simulink model "Closed_loop_Sim_2017a"  (R2017a)
settings: Solver=FixedStepAuto  StartTime=0.0  StopTime=400  FixedStep=tstep  RelTol=1e-3  EnableMultiTasking=on
InitFcn:
  | initSim;
values from neighbouring files (symbols this model uses):
  par = problem.data    [initSim.m]
undefined symbols (not defined in the file or in its folder): m, problem
settings Model: Creator=yn15  LastModifiedBy=Yuanb
settings OptimizationCC: LifeSpan=inf
settings DebuggingCC: SFUnexpectedBacktrackingDiag=warning  SFNoUnconditionalDefaultTransitionDiag=warning  SFExecutionAtInitializationDiag=none
settings GRTTargetCC: TargetLangStandard=C89/C90 (ANSI)
settings ConfigComp: CovMetricSettings=dw  CovHtmlReporting=on  CovSaveCumulativeToWorkspaceVar=on  CovSaveSingleToWorkspaceVar=on  CovExternalEMLEnable=off

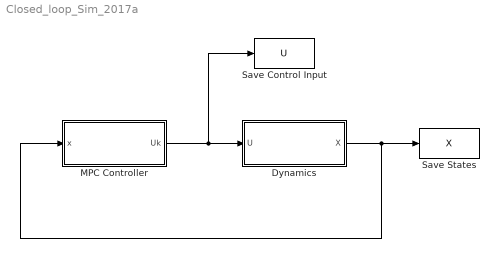
== system Closed_loop_Sim_2017a ==
  Dynamics : Subsystem
  "MPC Controller " : Subsystem
  Save Control Input : ToWorkspace  VariableName=U  SampleTime=-1
      settings: Save2DSignal=2-D array (concatenate along first dimension)
  Save States : ToWorkspace  VariableName=X  SampleTime=-1
  wires:
  "MPC Controller "/1(Uk) -> Dynamics/1(U), Save Control Input/1
  Dynamics/1(X) -> Save States/1, "MPC Controller "/1(x)

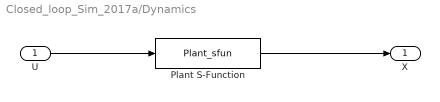
== system Closed_loop_Sim_2017a/Dynamics ==
  U : Inport
  Plant S-Function : S-Function  FunctionName=Plant_sfun  Parameters=par;problem.states.x0  SFunctionDeploymentMode=off  EnableBusSupport=off
  X : Outport
  wires:
  Plant S-Function/1 -> X/1
  U/1 -> Plant S-Function/1

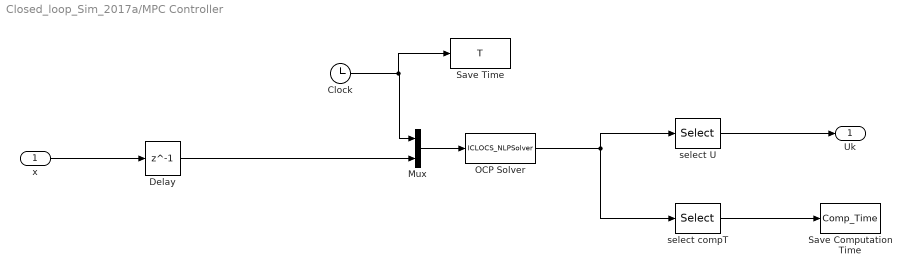
== system Closed_loop_Sim_2017a/MPC Controller  ==
  x : Inport
  Clock : Clock
  Delay : Delay  DelayLength=1  InitialCondition=[problem.states.x0]
  Mux : Mux  Inputs=2
  OCP Solver : MATLABFcn  MATLABFcn=ICLOCS_NLPSolver  OutputDimensions=m+2
  "Save Computation Time " : ToWorkspace  VariableName=Comp_Time  SampleTime=-1
      settings: Save2DSignal=2-D array (concatenate along first dimension)
  Save Time : ToWorkspace  VariableName=T  SampleTime=-1
      settings: Save2DSignal=2-D array (concatenate along first dimension)
  select U : Selector  IndexOptions=Index vector (dialog)  Indices=3:m+2  OutputSizes=1
  select compT : Selector  IndexOptions=Index vector (dialog)  Indices=2  OutputSizes=1
  Uk : Outport
  wires:
  select U/1 -> Uk/1
  x/1 -> Delay/1
  OCP Solver/1 -> select compT/1, select U/1
  Clock/1 -> Save Time/1, Mux/1
  Mux/1 -> OCP Solver/1
  Delay/1 -> Mux/2
  select compT/1 -> "Save Computation Time "/1
